simulink model "OptimizeAHRS"  (R2020a)
settings: Solver=FixedStepAuto  StartTime=0.0  StopTime=46.4  FixedStep=0.1  RelTol=1e-3
libraries: mspfiltlib x1
settings Model: OrderedModelArguments=off  Creator=AlexC  LastModifiedBy=AlexC

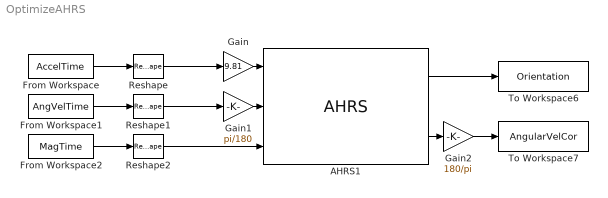
== system OptimizeAHRS ==
  AHRS1 : mspfiltlib/AHRS  DispRefFrame=NED  DecimationFactor=1  InitialProcessNoise=ahrsfilter.defaultProcessNoise  OrientationFormat=quaternion  SimulateUsing=Interpreted execution  AccelerometerNoise=a1  GyroscopeNoise=a2  MagnetometerNoise=a3  GyroscopeDriftNoise=a4  LinearAccelerationNoise=b1  MagneticDisturbanceNoise=b2  LinearAccelerationDecayFactor=b3  MagneticDisturbanceDecayFactor=b4  ExpectedMagneticFieldStrength=b5
      settings: SourceProductBaseCode=TF,NV
  From Workspace : FromWorkspace  VariableName=AccelTime  SampleTime=0.1
  From Workspace1 : FromWorkspace  VariableName=AngVelTime  SampleTime=0.1
  From Workspace2 : FromWorkspace  VariableName=MagTime  SampleTime=0.1
  Gain : Gain  Gain=9.81
  Gain1 : Gain  Gain=pi/180
  Gain2 : Gain  Gain=180/pi
  Reshape : Reshape  OutputDimensionality=Row vector (2-D)
  Reshape1 : Reshape  OutputDimensionality=Row vector (2-D)
  Reshape2 : Reshape  OutputDimensionality=Row vector (2-D)
  To Workspace6 : ToWorkspace  VariableName=Orientation  SampleTime=-1
      settings: Save2DSignal=2-D array (concatenate along first dimension)
  To Workspace7 : ToWorkspace  VariableName=AngularVelCor  SampleTime=-1
      settings: Save2DSignal=2-D array (concatenate along first dimension)
  wires:
  Gain/1 -> AHRS1/1
  AHRS1/1 -> To Workspace6/1
  Gain1/1 -> AHRS1/2
  AHRS1/2 -> Gain2/1
  Gain2/1 -> To Workspace7/1
  From Workspace/1 -> Reshape/1
  From Workspace1/1 -> Reshape1/1
  From Workspace2/1 -> Reshape2/1
  Reshape/1 -> Gain/1
  Reshape1/1 -> Gain1/1
  Reshape2/1 -> AHRS1/3
